simulink model "testmodel2"  (R2022b)
settings: Solver=FixedStepDiscrete  StartTime=0.0  StopTime=10.0  FixedStep=0.000001  RelTol=1e-3
settings Model: Creator=yll  LastModifiedBy=yll

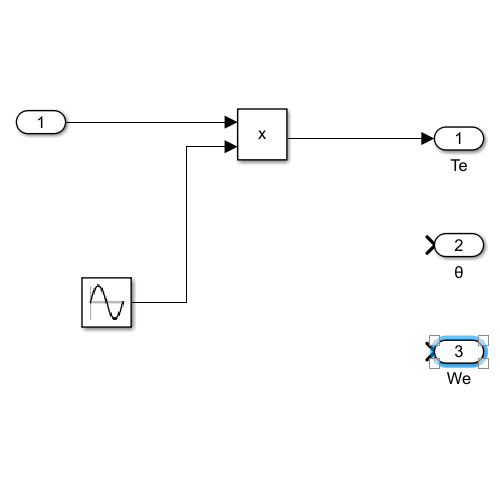
[thumbnail: Simulink's stored preview of the top-level diagram]
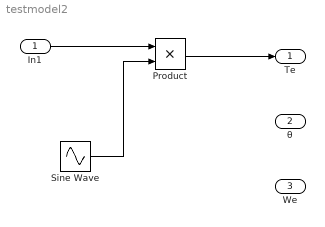
== system testmodel2 ==
  In1 : Inport
  Product : Product
  Sine Wave : Sin  Amplitude=2  Bias=90  SampleTime=0
  Te : Outport
  θ : Outport  Port=2
  We : Outport  Port=3
  wires:
  In1/1 -> Product/1
  Product/1 -> Te/1
  Sine Wave/1 -> Product/2
